simulink subsystem "KF_update"  (R2021a)
settings: Solver=VariableStepAuto  StartTime=0.0  StopTime=10.0  RelTol=1e-3
undefined symbols (not defined in the file): magnitude, str_std
libraries: dspmtrx3 x2, aerolibutil x1
settings Model: Creator=Laura  LastModifiedBy=Laura

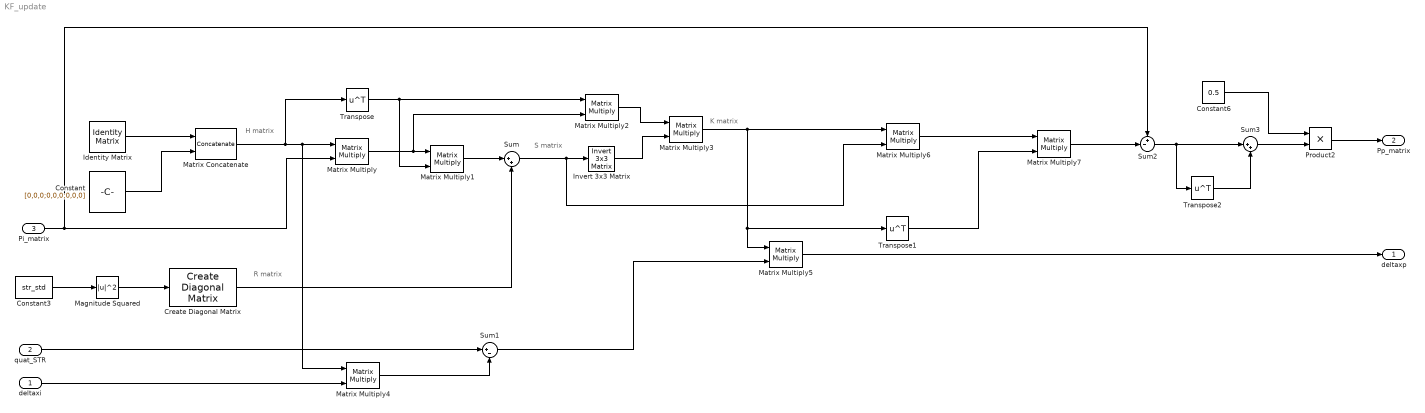
== system KF_update ==
  note: K matrix
  note: S matrix
  note: R matrix
  note: H matrix
  deltaxi : Inport
  quat_STR : Inport  Port=2
  Pi_matrix : Inport  Port=3
  Constant : Constant  Value=[0,0,0;0,0,0;0,0,0]
  Constant3 : Constant  Value=str_std
  Constant6 : Constant  Value=0.5
  Create Diagonal Matrix : dspmtrx3/Create Diagonal Matrix
      settings: SourceProductBaseCode=DS
  Identity Matrix : dspmtrx3/Identity Matrix  Inherit=off  N=3  Ts=1  dataType=double  isSigned=on  wordLen=16  udDataType=sfix(16)  fracBitsMode=Best precision  numFracBits=15  OutDataTypeStr=double  LastOutDataTypeStr=double
  Invert 3x3 Matrix : aerolibutil/Invert  3x3 Matrix
  Magnitude Squared : Math  Operator=magnitude^2  SaturateOnIntegerOverflow=on
  Matrix Concatenate : Concatenate  Mode=Multidimensional array  ConcatenateDimension=2
  Matrix Multiply{,1..7} (8 alike) : Product  Multiplication=Matrix(*)
  Product2 : Product
  Sum : Sum  Inputs=|++
  Sum1 : Sum  Inputs=|+-
  Sum2 : Sum  Inputs=+-|
  Sum3 : Sum  Inputs=|++
  Transpose : Math  Operator=transpose  SaturateOnIntegerOverflow=on
  Transpose1 : Math  Operator=transpose  SaturateOnIntegerOverflow=on
  Transpose2 : Math  Operator=transpose  SaturateOnIntegerOverflow=on
  deltaxp : Outport
  Pp_matrix : Outport  Port=2
  wires:
  Constant3/1 -> Magnitude Squared/1
  Magnitude Squared/1 -> Create Diagonal Matrix/1
  Identity Matrix/1 -> Matrix Concatenate/1
  Constant/1 -> Matrix Concatenate/2
  Matrix Concatenate/1 -> Transpose/1, Matrix Multiply4/1, Matrix Multiply/1
  Pi_matrix/1 -> Matrix Multiply/2, Sum2/1
  Transpose/1 -> Matrix Multiply2/1, Matrix Multiply1/2
  Create Diagonal Matrix/1 -> Sum/2
  Matrix Multiply1/1 -> Sum/1
  Sum/1 -> Invert 3x3 Matrix/1, Matrix Multiply6/2
  Matrix Multiply/1 -> Matrix Multiply2/2, Matrix Multiply1/1
  Matrix Multiply2/1 -> Matrix Multiply3/1
  Invert 3x3 Matrix/1 -> Matrix Multiply3/2
  quat_STR/1 -> Sum1/1
  deltaxi/1 -> Matrix Multiply4/2
  Matrix Multiply4/1 -> Sum1/2
  Sum1/1 -> Matrix Multiply5/2
  Matrix Multiply3/1 -> Transpose1/1, Matrix Multiply5/1, Matrix Multiply6/1
  Matrix Multiply5/1 -> deltaxp/1
  Matrix Multiply6/1 -> Matrix Multiply7/1
  Transpose1/1 -> Matrix Multiply7/2
  Matrix Multiply7/1 -> Sum2/2
  Sum2/1 -> Transpose2/1, Sum3/1
  Sum3/1 -> Product2/2
  Product2/1 -> Pp_matrix/1
  Constant6/1 -> Product2/1
  Transpose2/1 -> Sum3/2
